simulink model "BLDCM"  (R2022a)
settings: Solver=FixedStepDiscrete  StartTime=0.0  StopTime=1  FixedStep=0.000001  RelTol=1e-3
libraries: simulink x3, slpidlib x2, spsDCVoltageSourceLib x1, spsPermanentMagnetSynchronousMachineLib x1, spsTwoLevelConverterLib x1, spspowerguiLib x1
settings Model: Creator=solituder  LastModifiedBy=solituder

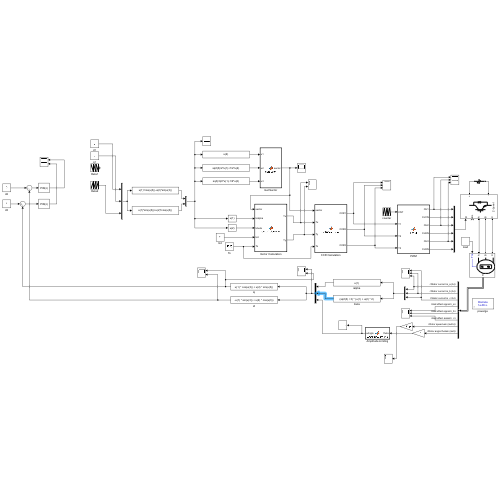
[thumbnail: Simulink's stored preview of the top-level diagram]
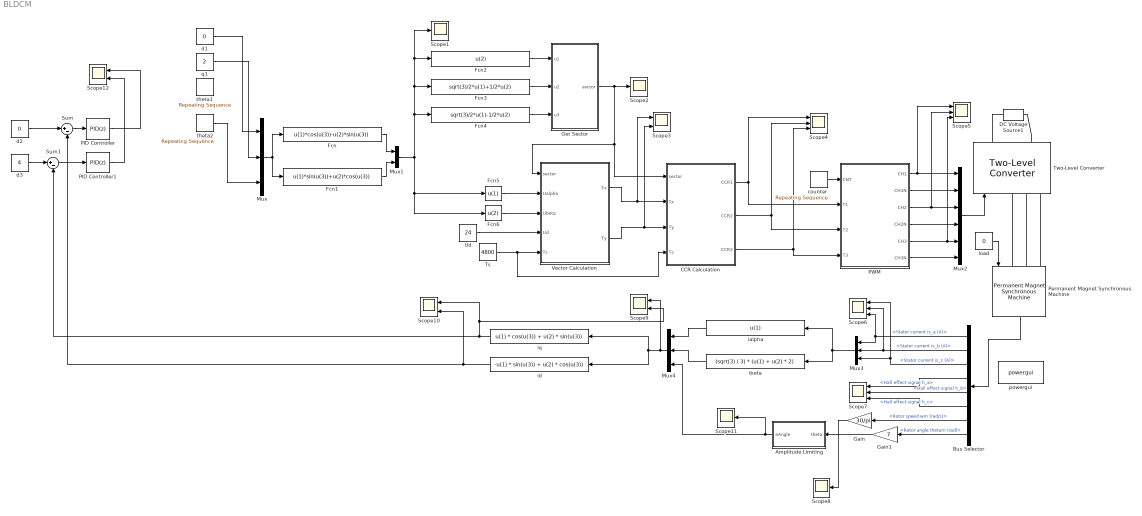
== system BLDCM ==
  Amplitude Limiting : MATLAB Function  TreatAsAtomicUnit=on
  Bus Selector : BusSelector  OutputSignals=Stator current is_a (A),Stator current is_b (A),Stator current is_c (A),Hall effect signal h_a,Hall effect signal h_b,Hall effect signal h_c,Rotor speed wm (rad/s),Rotor angle thetam (rad)
  CCR Calculation : MATLAB Function  TreatAsAtomicUnit=on
  DC Voltage Source1 : spsDCVoltageSourceLib/DC Voltage Source  Amplitude=100  Measurements=None
  Fcn : Fcn  Expr=u(1)*cos(u(3))-u(2)*sin(u(3))
  Fcn1 : Fcn  Expr=u(1)*sin(u(3))+u(2)*cos(u(3))
  Fcn2 : Fcn  Expr=u(2)
  Fcn3 : Fcn  Expr=sqrt(3)/2*u(1)+1/2*u(2)
  Fcn4 : Fcn  Expr=sqrt(3)/2*u(1)-1/2*u(2)
  Fcn5 : Fcn  Expr=u(1)
  Fcn6 : Fcn  Expr=u(2)
  Gain : Gain  Gain=30/pi
  Gain1 : Gain  Gain=7
  Get Sector : MATLAB Function  TreatAsAtomicUnit=on
  Mux : Mux  Inputs=3
  Mux1 : Mux  Inputs=2
  Mux2 : Mux  Inputs=6
  Mux3 : Mux  Inputs=3
  Mux4 : Mux  Inputs=3
  PID Controller : slpidlib/PID Controller  Controller=PID  Form=Ideal  TimeDomain=Discrete-time  UseExternalTs=off  SampleTime=-1  IntegratorMethod=Forward Euler  FilterMethod=Forward Euler  ControllerParametersSource=internal  P=1  I=1  UseKiTs=off  D=0  N=100  UseFilter=on  TunerSelectOption=Transfer Function Based (PID Tuner App)  InitialConditionSource=internal  InitialConditionForIntegrator=0  InitialConditionForFilter=0  DifferentiatorICPrevScaledInput=0  ExternalReset=none  TrackingMode=off  Kt=1  LimitOutput=off  SatLimitsSource=internal  UpperSaturationLimit=inf  LowerSaturationLimit=-inf  LinearizeAsGain=on  AntiWindupMode=none  Kb=1  POutMin=[]  POutMax=[]  IOutMin=[]  IOutMax=[]  DOutMin=[]  DOutMax=[]  NOutMin=[]  NOutMax=[]  SumOutMin=[]  SumOutMax=[]  SaturationOutMin=[]  SaturationOutMax=[]  PParamMin=[]  PParamMax=[]  IParamMin=[]  IParamMax=[]  DParamMin=[]  DParamMax=[]  NParamMin=[]  NParamMax=[]  KbParamMin=[]  KbParamMax=[]  KtParamMin=[]  KtParamMax=[]  KbOutMin=[]  KbOutMax=[]  KtOutMin=[]  KtOutMax=[]  IntegratorOutMin=[]  IntegratorOutMax=[]  FilterOutMin=[]  FilterOutMax=[]  SumI1OutMin=[]  SumI1OutMax=[]  SumI2OutMin=[]  SumI2OutMax=[]  SumI3OutMin=[]  SumI3OutMax=[]  SumI4OutMin=[]  SumI4OutMax=[]  SumDOutMin=[]  SumDOutMax=[]  DifferentiatorOutMin=[]  DifferentiatorOutMax=[]  FilterDiffOutCoefMin=[]  FilterDiffOutCoefMax=[]  ReciprocalOutMin=[]  ReciprocalOutMax=[]  SumDenOutMin=[]  SumDenOutMax=[]  SumNumOutMin=[]  SumNumOutMax=[]  DivideOutMin=[]  DivideOutMax=[]  UdiffTsProdOutMin=[]  UdiffTsProdOutMax=[]  NTsProdOutMin=[]  NTsProdOutMax=[]  UintegralTsProdOutMin=[]  UintegralTsProdOutMax=[]  UngainTsProdOutMin=[]  UngainTsProdOutMax=[]  IntegratorContinuousStateAttributes=''  IntegratorStateMustResolveToSignalObject=off  IntegratorRTWStateStorageClass=Auto  FilterContinuousStateAttributes=''  FilterStateMustResolveToSignalObject=off  FilterRTWStateStorageClass=Auto  ParallelPVariant=Passthrough  IdealPVariant=InternalParameters  IVariant=InternalParameters  DVariant=InternalParameters  IntegratorVariant=Discrete  SatVariant=Disabled  AWVariant=Passthrough  PCopyVariant=Disabled  TRVariant=Disabled  FdbkBlocksVariant=Forward  IdealPFdbkVariant=Disabled  SatFdbkVariant=Disabled  DerivativeFilterVariant=ForwardEulerFilter  NVariant=InternalParameters  NCopyVariant=Disabled  FilterICVariant=InternalICsFilter  IntegratorICVariant=InternalICs  ExternalResetVariant=Disabled  TRSumVariant=Passthrough  SumFdbkVariant=Disabled  SumVariant=Sum_PID  TsampFilterVariant=InternalTs  TsampNgainVariant=Passthrough  TsampIntegralVariant=Passthrough  ExternalSaturationOutDataTypeStr=Inherit: Same as second input  aMode=0
  PID Controller1 : slpidlib/PID Controller  Controller=PID  Form=Ideal  TimeDomain=Discrete-time  UseExternalTs=off  SampleTime=-1  IntegratorMethod=Forward Euler  FilterMethod=Forward Euler  ControllerParametersSource=internal  P=3  I=2  UseKiTs=off  D=9  N=100  UseFilter=on  TunerSelectOption=Transfer Function Based (PID Tuner App)  InitialConditionSource=internal  InitialConditionForIntegrator=0  InitialConditionForFilter=0  DifferentiatorICPrevScaledInput=0  ExternalReset=none  TrackingMode=off  Kt=1  LimitOutput=off  SatLimitsSource=internal  UpperSaturationLimit=inf  LowerSaturationLimit=-inf  LinearizeAsGain=on  AntiWindupMode=none  Kb=1  POutMin=[]  POutMax=[]  IOutMin=[]  IOutMax=[]  DOutMin=[]  DOutMax=[]  NOutMin=[]  NOutMax=[]  SumOutMin=[]  SumOutMax=[]  SaturationOutMin=[]  SaturationOutMax=[]  PParamMin=[]  PParamMax=[]  IParamMin=[]  IParamMax=[]  DParamMin=[]  DParamMax=[]  NParamMin=[]  NParamMax=[]  KbParamMin=[]  KbParamMax=[]  KtParamMin=[]  KtParamMax=[]  KbOutMin=[]  KbOutMax=[]  KtOutMin=[]  KtOutMax=[]  IntegratorOutMin=[]  IntegratorOutMax=[]  FilterOutMin=[]  FilterOutMax=[]  SumI1OutMin=[]  SumI1OutMax=[]  SumI2OutMin=[]  SumI2OutMax=[]  SumI3OutMin=[]  SumI3OutMax=[]  SumI4OutMin=[]  SumI4OutMax=[]  SumDOutMin=[]  SumDOutMax=[]  DifferentiatorOutMin=[]  DifferentiatorOutMax=[]  FilterDiffOutCoefMin=[]  FilterDiffOutCoefMax=[]  ReciprocalOutMin=[]  ReciprocalOutMax=[]  SumDenOutMin=[]  SumDenOutMax=[]  SumNumOutMin=[]  SumNumOutMax=[]  DivideOutMin=[]  DivideOutMax=[]  UdiffTsProdOutMin=[]  UdiffTsProdOutMax=[]  NTsProdOutMin=[]  NTsProdOutMax=[]  UintegralTsProdOutMin=[]  UintegralTsProdOutMax=[]  UngainTsProdOutMin=[]  UngainTsProdOutMax=[]  IntegratorContinuousStateAttributes=''  IntegratorStateMustResolveToSignalObject=off  IntegratorRTWStateStorageClass=Auto  FilterContinuousStateAttributes=''  FilterStateMustResolveToSignalObject=off  FilterRTWStateStorageClass=Auto  ParallelPVariant=Passthrough  IdealPVariant=InternalParameters  IVariant=InternalParameters  DVariant=InternalParameters  IntegratorVariant=Discrete  SatVariant=Disabled  AWVariant=Passthrough  PCopyVariant=Disabled  TRVariant=Disabled  FdbkBlocksVariant=Forward  IdealPFdbkVariant=Disabled  SatFdbkVariant=Disabled  DerivativeFilterVariant=ForwardEulerFilter  NVariant=InternalParameters  NCopyVariant=Disabled  FilterICVariant=InternalICsFilter  IntegratorICVariant=InternalICs  ExternalResetVariant=Disabled  TRSumVariant=Passthrough  SumFdbkVariant=Disabled  SumVariant=Sum_PID  TsampFilterVariant=InternalTs  TsampNgainVariant=Passthrough  TsampIntegralVariant=Passthrough  ExternalSaturationOutDataTypeStr=Inherit: Same as second input  aMode=0
  PWM : MATLAB Function  TreatAsAtomicUnit=on
  Permanent Magnet Synchronous Machine : spsPermanentMagnetSynchronousMachineLib/Permanent Magnet Synchronous Machine  NbPhases=3  FluxDistribution=Sinusoidal  RotorType=Round  MechanicalLoad=Torque Tm  PresetModel=No  ShowDetailedParameters=on  MeasurementBus=off  Resistance=0.0485  Inductance=8.5e-3  dqInductances=[8.5e-3,8.5e-3]  La=0.000395  MachineConstant=Flux linkage established by magnets (V.s)  Flux=0.1194  VoltageCst=151.5974  TorqueCst=1.2537  Flat=120  Mechanical=[0.0027 0.0004924 7 0]  PolePairs=4  InitialConditions=[0,0, 0,0]  InitialConditions5ph=[0 0 0 0 0 0]  RefAngle=Aligned with phase A axis (original Park)  IterativeDiscreteModel=Trapezoidal non iterative  TsBlock=-1  TsPowergui=0
  Scope{1..2,8,11} (4 alike) : Scope
  Scope{3,9..10,12} (4 alike) : Scope  NumInputPorts=2
  Scope{4..7} (4 alike) : Scope  NumInputPorts=3
  Sum : Sum  Inputs=|+-
  Sum1 : Sum  Inputs=|+-
  Ts : Constant  Value=4800
  Two-Level Converter : spsTwoLevelConverterLib/Two-Level Converter  ModelType=Switching devices  Ron=1e-3  Rs=1e6  Cs=inf  Vforward=[0,0]  Ron_Diode=1e-3  Rs_Diode=1e6  Cs_Diode=inf  Vf_Diode=1e-3  Rs_CurrentSource=inf  Ron_ACsource=1e-3
      settings: SourceProductBaseCode=PS
  Ud : Constant  Value=24
  Vector Calculation : MATLAB Function  TreatAsAtomicUnit=on
  counter : simulink/Sources/Repeating Sequence  rep_seq_t=[0 0.00006667 0.00013334]  rep_seq_y=[0 4800 0]
  d1 : Constant  Value=0
  d2 : Constant  Value=0
  d3 : Constant  Value=4
  ialpha : Fcn  Expr=u(1)
  ibeta : Fcn  Expr=(sqrt(3) / 3) * (u(1) + u(2) * 2)
  id : Fcn  Expr=-u(1) * sin(u(3)) + u(2) * cos(u(3))
  iq : Fcn  Expr=u(1) * cos(u(3)) + u(2) * sin(u(3))
  load : Constant  Value=0
  powergui : spspowerguiLib/powergui  Priority=1  SimulationMode=Discrete  SampleTime=0.000001  frequency=60  Iterations=50  frequencyindice=0  Pbase=100e6  ErrMax=1e-4  UnitsV=kV  UnitsW=MW  buscounter=0  FunctionMessages=off  echomessages=off  EnableUseOfTLC=off  CurrentSourceSwitches=off  DisableSnubberDevices=off  DisableRonSwitches=off  DisableVfSwitches=off  DisplayEquations=off  AutomaticDiscreteSolvers=off  SolverType=Tustin/Backward Euler (TBE)  Interpol=off  ExternalGateDelay=off  methode=off  Ts=100  x0status=blocks  SPID=on  SwTol=0  HookPort=off  NonlinearTolerance=1e-4  nMaxIteration=100  ContinueOnMaxIteration=off  RestoreLinks=warning  ResistiveCurrentMeasurement=off  Frange=[0:2:500]  Ylog=off  Xlog=on  ShowGrid=off  save=off  variable=ZData  structure=0  ZoomFFT=off  StartTime=0.0  cycles=1  DisplayStyle=1  fundamental=60  FreqAxis=off  MaxFrequency=1000  frequencyindicesteady=1  RmsSteady=1  display=off
  q1 : Constant  Value=2
  theta1 : simulink/Sources/Repeating Sequence  rep_seq_t=[0 0.1]  rep_seq_y=[2*pi 0]
  theta2 : simulink/Sources/Repeating Sequence  rep_seq_t=[0 0.1]  rep_seq_y=[0 2*pi]
  wires:
  Fcn/1 -> Mux1/1
  Fcn1/1 -> Mux1/2
  Mux1/1 -> Fcn6/1, Fcn5/1, Fcn3/1, Scope1/1, Fcn2/1, Fcn4/1
  Get Sector/1(sector) -> CCR Calculation/1(sector), Vector Calculation/1(sector), Scope2/1
  Fcn2/1 -> Get Sector/1(u1)
  Fcn3/1 -> Get Sector/2(u2)
  Fcn4/1 -> Get Sector/3(u3)
  Fcn5/1 -> Vector Calculation/2(Ualpha)
  Fcn6/1 -> Vector Calculation/3(Ubeta)
  Ud/1 -> Vector Calculation/4(Ud)
  Ts/1 -> Vector Calculation/5(Ts), CCR Calculation/4(Ts)
  Vector Calculation/1(Tx) -> Scope3/1, CCR Calculation/2(Tx)
  Vector Calculation/2(Ty) -> Scope3/2, CCR Calculation/3(Ty)
  CCR Calculation/1(CCR1) -> PWM/2(T1), Scope4/1
  CCR Calculation/2(CCR2) -> PWM/3(T2), Scope4/2
  CCR Calculation/3(CCR3) -> PWM/4(T3), Scope4/3
  counter/1 -> PWM/1(CNT)
  PWM/3(CH2) -> Mux2/3, Scope5/2
  PWM/4(CH2N) -> Mux2/4
  PWM/5(CH3) -> Scope5/3, Mux2/5
  PWM/6(CH3N) -> Mux2/6
  PWM/1(CH1) -> Scope5/1, Mux2/1
  PWM/2(CH1N) -> Mux2/2
  Mux2/1 -> Two-Level Converter/1
  load/1 -> Permanent Magnet Synchronous Machine/1
  Permanent Magnet Synchronous Machine/1 -> Bus Selector/1
  Bus Selector/4 -> Scope7/1  "<Hall effect signal h_a>"
  Bus Selector/5 -> Scope7/2  "<Hall effect signal h_b>"
  Bus Selector/6 -> Scope7/3  "<Hall effect signal h_c>"
  Bus Selector/3 -> Scope6/1, Mux3/3  "<Stator current is_c (A)>"
  Bus Selector/2 -> Scope6/2, Mux3/2  "<Stator current is_b (A)>"
  Bus Selector/1 -> Mux3/1, Scope6/3  "<Stator current is_a (A)>"
  Bus Selector/7 -> Gain/1  "<Rotor speed wm (rad/s)>"
  Mux4/1 -> Scope9/1, iq/1, id/1
  Gain/1 -> Scope8/1
  Mux/1 -> Fcn1/1, Fcn/1
  Bus Selector/8 -> Gain1/1  "<Rotor angle thetam (rad)>"
  iq/1 -> Sum1/2, Scope9/2, Scope10/1
  id/1 -> Sum/2, Scope10/2
  Gain1/1 -> Amplitude Limiting/1(theta)
  Amplitude Limiting/1(eAngle) -> Mux4/3, Scope11/1
  d2/1 -> Sum/1
  d3/1 -> Sum1/1
  Sum1/1 -> PID Controller1/1
  Sum/1 -> PID Controller/1
  PID Controller1/1 -> Scope12/2
  PID Controller/1 -> Scope12/1
  q1/1 -> Mux/2
  d1/1 -> Mux/1
  theta2/1 -> Mux/3
  Mux3/1 -> ialpha/1, ibeta/1
  ialpha/1 -> Mux4/1
  ibeta/1 -> Mux4/2
  connections:
  Two-Level Converter/RConn1 -- DC Voltage Source1/RConn1
  Two-Level Converter/RConn2 -- DC Voltage Source1/LConn1
  Permanent Magnet Synchronous Machine/LConn2 -- Two-Level Converter/LConn2
  Permanent Magnet Synchronous Machine/LConn3 -- Two-Level Converter/LConn3
  Permanent Magnet Synchronous Machine/LConn1 -- Two-Level Converter/LConn1

== matlab function BLDCM/Vector Calculation ==
  data: sector input; Tx output; Ualpha input; Ubeta input; Ud input; Ts input; Ty output
function [Tx, Ty] = sectorCalculation(sector, Ualpha, Ubeta, Ud, Ts)

Tx = double(0);
Ty = double(0);

Ux = (sqrt(3) * Ts) / Ud * Ubeta;
Uy = (sqrt(3) * Ts) / Ud * ((sqrt(3) / 2) * Ualpha - (1 / 2) * Ubeta);
Uz = (sqrt(3) * Ts) / Ud * ((sqrt(3) / 2) * Ualpha + (1 / 2) * Ubeta);

if(sector == 1)
    Tx = Uy;
    Ty = Ux;
end

if(sector == 2)
    Tx = -Uy;
    Ty = Uz;
end

if(sector == 3)
    Tx = Ux;
    Ty = -Uz;
end

if(sector == 4)
    Tx = -Ux;
    Ty = -Uy;
end

if(sector == 5)
    Tx = -Uz;
    Ty = Uy;
end

if(sector == 6)
    Tx = Uz;
    Ty = -Ux;
end

== matlab function BLDCM/Get Sector ==
  data: u1 input; sector output; u2 input; u3 input
function sector = getSector(u1, u2, u3)

sector = uint8(3);

if(u2 > 0)
    sector = sector - 1;
end
if(u3 > 0)
    sector = sector - 1;
end
if(u1 < 0)
    sector = 7 - sector;
end

== matlab function BLDCM/CCR Calculation ==
  data: sector input; CCR1 output; Tx input; Ty input; Ts input; CCR2 output; CCR3 output
function [CCR1, CCR2, CCR3] = CCRCalculation(sector, Tx, Ty, Ts)

CCR1 = double(0);
CCR2 = double(0);
CCR3 = double(0);

Ttemp = Tx + Ty;
if(Ttemp > Ts)
    Tx = Tx / Ttemp * Ts;
    Ty = Ty / Ttemp * Ts;
end

Tc = (Ts - Ttemp) / 2;
Tb = Tc + Ty;
Ta = Tb + Tx;

switch(sector)
    case 1
		CCR1 = Ta;
		CCR2 = Tb;
		CCR3 = Tc; 
    case 2
		CCR1 = Tb;
		CCR2 = Ta;
		CCR3 = Tc;
	case 3
		CCR1 = Tc;
		CCR2 = Ta;
		CCR3 = Tb;
	case 4
		CCR1 = Tc;
		CCR2 = Tb;
		CCR3 = Ta;
    case 5
		CCR1 = Tb;
		CCR2 = Tc;
		CCR3 = Ta;
	case 6
		CCR1 = Ta;
		CCR2 = Tc;
		CCR3 = Tb;
end

== matlab function BLDCM/PWM ==
  data: CNT input; T1 input; CH1 output; T2 input; T3 input; CH1N output; CH2 output; CH2N output; CH3 output; CH3N output
function [CH1, CH1N, CH2, CH2N, CH3, CH3N] = PWM(CNT, T1, T2, T3)

if(CNT < T1)
    CH1 = 0;
    CH1N = 1;
else
    CH1 = 1;
    CH1N = 0;    
end

if(CNT < T2)
    CH2 = 0;
    CH2N = 1;
else
    CH2 = 1;
    CH2N = 0; 
end

if(CNT < T3)
    CH3 = 0;
    CH3N = 1;
else
    CH3 = 1;
    CH3N = 0; 
end

== matlab function BLDCM/Amplitude Limiting ==
  data: theta input; eAngle output
function eAngle =  amplitudeLimiting(theta)

eAngle = mod(theta, 6.28);
